simulink model "example_of_temperature_sensor"  (R2021a)
settings: Solver=VariableStepAuto  StartTime=0.0  StopTime=100  RelTol=1e-3
libraries: simulink x5
settings Model: Creator=YasserNet  LastModifiedBy=YasserNet

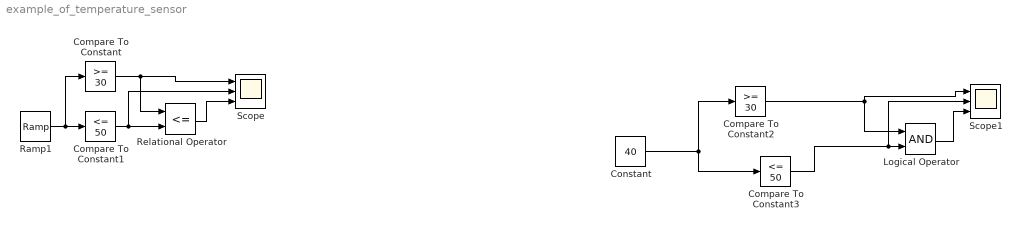
== system example_of_temperature_sensor ==
  Compare To Constant : simulink/Logic and Bit Operations/Compare To Constant  relop=>=  const=30  OutDataTypeStr=boolean
  Compare To Constant1 : simulink/Logic and Bit Operations/Compare To Constant  relop=<=  const=50  OutDataTypeStr=boolean
  Compare To Constant2 : simulink/Logic and Bit Operations/Compare To Constant  relop=>=  const=30  OutDataTypeStr=boolean
  Compare To Constant3 : simulink/Logic and Bit Operations/Compare To Constant  relop=<=  const=50  OutDataTypeStr=boolean
  Constant : Constant  Value=40
  Logical Operator : Logic  AllPortsSameDT=off  OutDataTypeStr=boolean
  Ramp1 : simulink/Sources/Ramp  slope=1  start=20  InitialOutput=30
  Relational Operator : RelationalOperator  Operator=<=  OutDataTypeStr=boolean  RndMeth=Simplest
  Scope : Scope  NumInputPorts=3
  Scope1 : Scope  NumInputPorts=3
  wires:
  Logical Operator/1 -> Scope1/3
  Compare To Constant1/1 -> Relational Operator/2, Scope/2
  Constant/1 -> Compare To Constant3/1, Compare To Constant2/1
  Compare To Constant2/1 -> Scope1/1, Logical Operator/1
  Ramp1/1 -> Compare To Constant1/1, Compare To Constant/1
  Compare To Constant3/1 -> Logical Operator/2, Scope1/2
  Compare To Constant/1 -> Relational Operator/1, Scope/1
  Relational Operator/1 -> Scope/3
